simulink model "StairCaseWaveGenerator"  (R2020b)
settings: Solver=VariableStepAuto  StartTime=0.0  StopTime=1  FixedStep=1  MaxStep=0.01  RelTol=1e-3
settings Model: Creator=99003759  LastModifiedBy=99003759

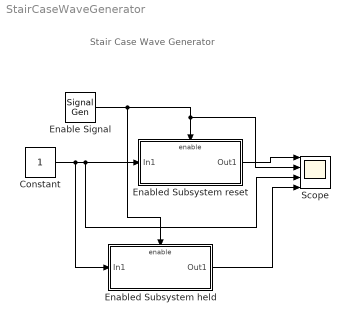
== system StairCaseWaveGenerator ==
  note: Stair Case Wave Generator
  Constant : Constant
  Enable Signal : SignalGenerator  WaveForm=square  Frequency=3
  Enabled Subsystem held : Subsystem  TreatAsAtomicUnit=on
  Enabled Subsystem reset : Subsystem  TreatAsAtomicUnit=on
  Scope : Scope  NumInputPorts=4
  wires:
  Enabled Subsystem reset/1(Out1) -> Scope/1
  Constant/1 -> Enabled Subsystem held/1(In1), Scope/3, Enabled Subsystem reset/1(In1)
  Enable Signal/1 -> Enabled Subsystem held/Enable, Scope/2, Enabled Subsystem reset/Enable
  Enabled Subsystem held/1(Out1) -> Scope/4

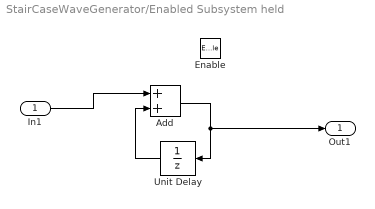
== system StairCaseWaveGenerator/Enabled Subsystem held ==
  In1 : Inport
  Enable : EnablePort
  Add : Sum
  Unit Delay : UnitDelay  SampleTime=-1  HasFrameUpgradeWarning=on
  Out1 : Outport
  wires:
  Add/1 -> Unit Delay/1, Out1/1
  In1/1 -> Add/1
  Unit Delay/1 -> Add/2

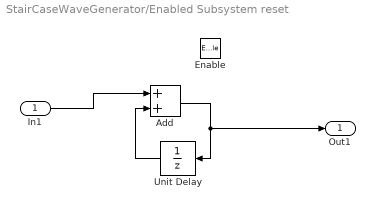
== system StairCaseWaveGenerator/Enabled Subsystem reset ==
  In1 : Inport
  Enable : EnablePort  StatesWhenEnabling=reset
  Add : Sum
  Unit Delay : UnitDelay  SampleTime=-1  HasFrameUpgradeWarning=on
  Out1 : Outport
  wires:
  Unit Delay/1 -> Add/2
  In1/1 -> Add/1
  Add/1 -> Out1/1, Unit Delay/1
